simulink model "bus_mess_test"  (Simulink 8.4)
settings: Solver=VariableStepDiscrete  StartTime=0.0  StopTime=0  MaxStep=1  RelTol=1e-3
undefined symbols (not defined in the file or in its folder): a2, a3
settings Model: Creator=arnaud  LastModifiedBy=arnaud
settings DataIOCC: SaveFormat=Structure  SignalLoggingSaveFormat=Dataset
settings OptimizationCC: ExpressionDepthLimit=128
settings DebuggingCC: UnderspecifiedInitializationDetection=Simplified  MergeDetectMultiDrivingBlocksExec=error  FcnCallInpInsideContextMsg=EnableAllAsError  StateNameClashWarn=none
settings GRTTargetCC: CombineOutputUpdateFcns=on  GRTInterface=off

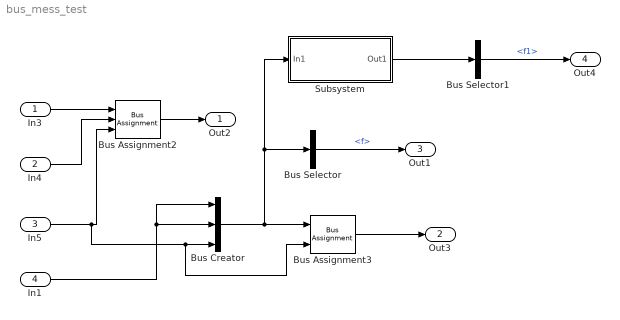
== system bus_mess_test ==
  In3 : Inport  OutDataTypeStr=Bus: BusA  BusOutputAsStruct=on
  In4 : Inport  Port=2  OutDataTypeStr=boolean
  In5 : Inport  Port=3  OutDataTypeStr=double
  In1 : Inport  Port=4  OutDataTypeStr=double
  Bus Assignment2 : BusAssignment  AssignedSignals=a2,a3
  Bus Assignment3 : BusAssignment  AssignedSignals=f1
  Bus Creator : BusCreator  Inputs=3  OutDataTypeStr=Bus: BusUnif3
      settings: InheritFromInputs=off
  Bus Selector : BusSelector  OutputSignals=f
  Bus Selector1 : BusSelector  OutputSignals=f1
  Subsystem : Subsystem  TreatAsAtomicUnit=on
  Out2 : Outport
  Out3 : Outport  Port=2
  Out1 : Outport  Port=3
  Out4 : Outport  Port=4
  wires:
  In3/1 -> Bus Assignment2/1
  In4/1 -> Bus Assignment2/2
  Bus Assignment2/1 -> Out2/1
  In5/1 -> Bus Assignment3/2, Bus Creator/3, Bus Assignment2/3
  Bus Assignment3/1 -> Out3/1
  Bus Selector/1 -> Out1/1  "<f>"
  In1/1 -> Bus Creator/2, Bus Creator/1
  Bus Selector1/1 -> Out4/1  "<f1>"
  Bus Creator/1 -> Subsystem/1(In1), Bus Selector/1, Bus Assignment3/1
  Subsystem/1(Out1) -> Bus Selector1/1

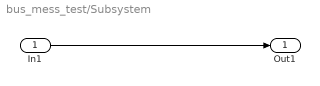
== system bus_mess_test/Subsystem ==
  In1 : Inport
  Out1 : Outport
  wires:
  In1/1 -> Out1/1
